simulink subsystem "rateLimiter"  (R2026a)
settings: Solver=VariableStepAuto
libraries: simulink x1, sl_discontinuities x1
settings Model: Creator=maxhu  LastModifiedBy=maxhu

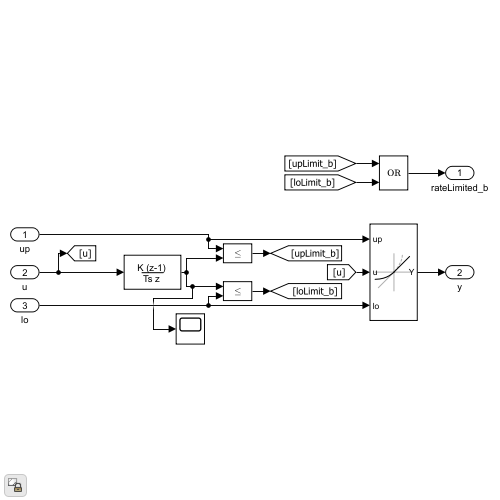
[thumbnail: Simulink's stored preview of the top-level diagram]
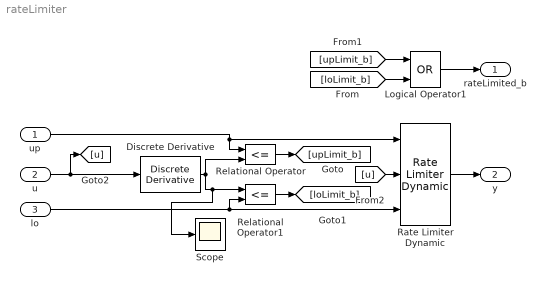
== system rateLimiter ==
  up : Inport
  u : Inport  Port=2
  lo : Inport  Port=3
  Discrete Derivative : simulink/Discrete/Discrete Derivative  gainval=1.0  ICPrevScaledInput=0.0  OutMin=[]  OutMax=[]  OutDataType=fixdt(1, 16)  OutScaling=2^-10  DoSatur=off
  Logical Operator1 : Logic  Operator=OR  AllPortsSameDT=off  OutDataTypeStr=boolean
  Rate Limiter Dynamic : sl_discontinuities/Rate Limiter Dynamic
  Relational Operator : RelationalOperator  Operator=<=  OutDataTypeStr=boolean  RndMeth=Simplest  InputSameDT=off
  Relational Operator1 : RelationalOperator  Operator=<=  OutDataTypeStr=boolean  RndMeth=Simplest  InputSameDT=off
  Scope : Scope
      settings: ActiveDisplayYMinimum=-1  ActiveDisplayYMaximum=1  DataLoggingVariableName=ScopeData5
  rateLimited_b : Outport
  y : Outport  Port=2
  wires:
  up/1 -> Relational Operator/1, Rate Limiter Dynamic/1
  lo/1 -> Relational Operator1/2, Rate Limiter Dynamic/3
  Rate Limiter Dynamic/1 -> y/1
  Logical Operator1/1 -> rateLimited_b/1
  Relational Operator/1 -> [upLimit_b]
  Relational Operator1/1 -> [loLimit_b]
  [upLimit_b] -> Logical Operator1/1
  [loLimit_b] -> Logical Operator1/2
  Discrete Derivative/1 -> Relational Operator/2, Relational Operator1/1, Scope/1
  u/1 -> Discrete Derivative/1, [u]
  [u] -> Rate Limiter Dynamic/2
